simulink model "sautrador"  (R2022a)
settings: Solver=VariableStepAuto  StartTime=0.0  StopTime=20  RelTol=1e-3
settings Model: Creator=souza  LastModifiedBy=souza

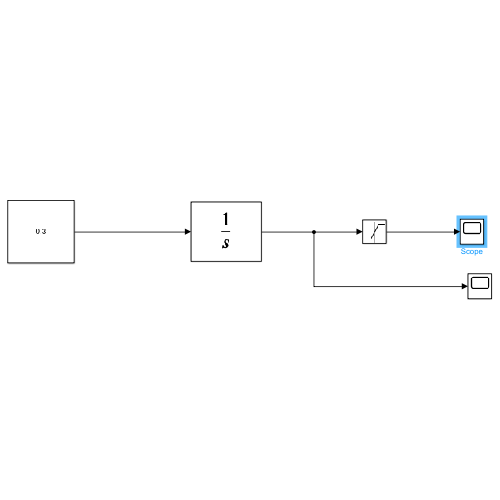
[thumbnail: Simulink's stored preview of the top-level diagram]
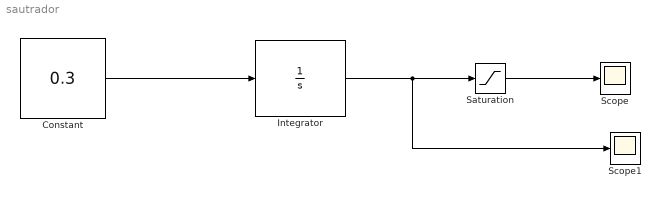
== system sautrador ==
  Constant : Constant  Value=0.3
  Integrator : Integrator  InitialCondition=0.5
  Saturation : Saturate  UpperLimit=1  LowerLimit=-1
  Scope : Scope
  Scope1 : Scope
  wires:
  Integrator/1 -> Scope1/1, Saturation/1
  Constant/1 -> Integrator/1
  Saturation/1 -> Scope/1
